simulink model "follower_v4"  (R2024a)
settings: Solver=VariableStepAuto  StartTime=0.0  StopTime=inf  RelTol=1e-6
values from neighbouring files (symbols this model uses):
  consigne = 0.6    [main.m]
undefined symbols (not defined in the file or in its folder): linear
libraries: ros2lib x5, slpidlib x1
settings Model: Creator=eswarm  LastModifiedBy=eswarm

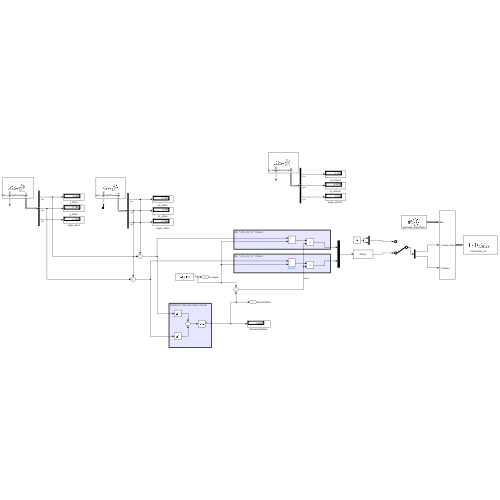
[thumbnail: Simulink's stored preview of the top-level diagram]
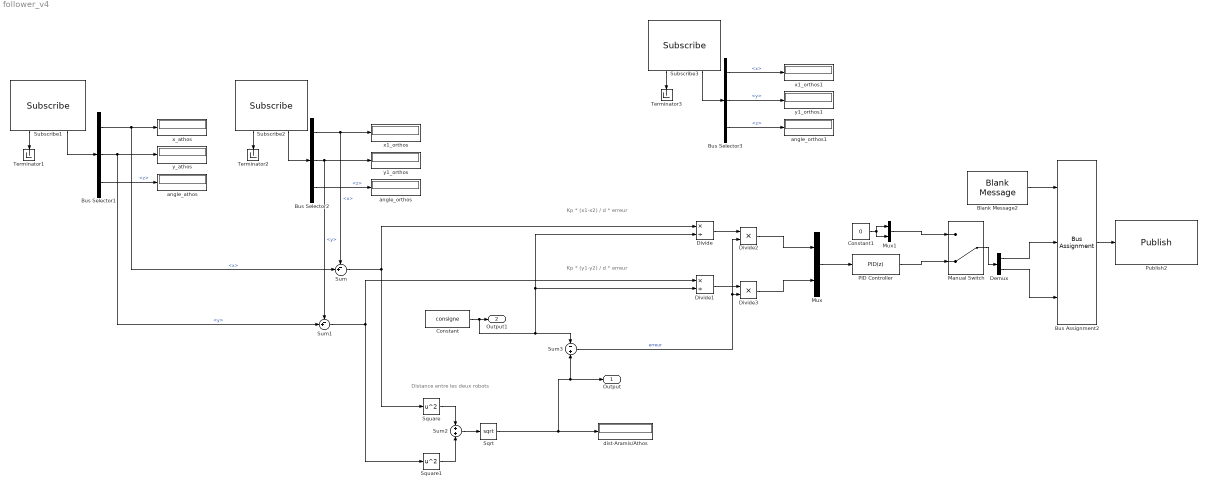
== system follower_v4 ==
  note: Distance entre les deux robots
  note: Kp * (x1-x2) / d * erreur
  note: Kp * (y1-y2) / d * erreur
  Blank Message2 : ros2lib/Blank Message  messageClass=Message  entityType=geometry_msgs/Twist  messageType=geometry_msgs/Twist  SampleTime=0.1
  Bus Assignment2 : BusAssignment  AssignedSignals=linear.x,linear.y
  Bus Selector1 : BusSelector  OutputSignals=pose.position.x,pose.position.y,pose.orientation.z
  Bus Selector2 : BusSelector  OutputSignals=pose.position.x,pose.position.y,pose.orientation.z
  Bus Selector3 : BusSelector  OutputSignals=pose.position.x,pose.position.y,pose.orientation.z
  Constant : Constant  Value=consigne
  Constant1 : Constant  Value=0
  Demux : Demux  Outputs=2
  Divide : Product  Inputs=*/  RndMeth=Zero  SaturateOnIntegerOverflow=on
  Divide1 : Product  Inputs=*/  RndMeth=Zero  SaturateOnIntegerOverflow=on
  Divide2 : Product  Inputs=**  RndMeth=Zero  SaturateOnIntegerOverflow=on
  Divide3 : Product  Inputs=**  RndMeth=Zero  SaturateOnIntegerOverflow=on
  Manual Switch : ManualSwitch  CurrentSetting=0
  Mux : Mux  Inputs=2
  Mux1 : Mux  Inputs=2
  PID Controller : slpidlib/PID Controller  Controller=PID  Form=Ideal  TimeDomain=Discrete-time  UseExternalTs=off  SampleTime=0.1  IntegratorMethod=Forward Euler  FilterMethod=Forward Euler  ControllerParametersSource=internal  P=0.5  I=0  UseKiTs=off  D=0  UseExternalDerivativeSource=off  N=100  UseFilter=on  TunerSelectOption=Transfer Function Based (PID Tuner App)  InitialConditionSource=internal  InitialConditionForIntegrator=0  InitialConditionForFilter=0  DifferentiatorICPrevScaledInput=0  ExternalReset=none  TrackingMode=off  Kt=1  LimitOutput=off  SatLimitsSource=internal  UpperSaturationLimit=inf  LowerSaturationLimit=-inf  LinearizeAsGain=on  AntiWindupMode=none  Kb=1  LimitIntegrator=off  UpperIntegratorSaturationLimit=inf  LowerIntegratorSaturationLimit=-inf  POutMin=[]  POutMax=[]  IOutMin=[]  IOutMax=[]  DOutMin=[]  DOutMax=[]  NOutMin=[]  NOutMax=[]  SumOutMin=[]  SumOutMax=[]  SaturationOutMin=[]  SaturationOutMax=[]  PParamMin=[]  PParamMax=[]  IParamMin=[]  IParamMax=[]  DParamMin=[]  DParamMax=[]  NParamMin=[]  NParamMax=[]  KbParamMin=[]  KbParamMax=[]  KtParamMin=[]  KtParamMax=[]  KbOutMin=[]  KbOutMax=[]  KtOutMin=[]  KtOutMax=[]  IntegratorOutMin=[]  IntegratorOutMax=[]  FilterOutMin=[]  FilterOutMax=[]  SumI1OutMin=[]  SumI1OutMax=[]  SumI2OutMin=[]  SumI2OutMax=[]  SumI3OutMin=[]  SumI3OutMax=[]  SumI4OutMin=[]  SumI4OutMax=[]  SumDOutMin=[]  SumDOutMax=[]  DifferentiatorOutMin=[]  DifferentiatorOutMax=[]  FilterDiffOutCoefMin=[]  FilterDiffOutCoefMax=[]  ReciprocalOutMin=[]  ReciprocalOutMax=[]  SumDenOutMin=[]  SumDenOutMax=[]  SumNumOutMin=[]  SumNumOutMax=[]  DivideOutMin=[]  DivideOutMax=[]  UdiffTsProdOutMin=[]  UdiffTsProdOutMax=[]  NTsProdOutMin=[]  NTsProdOutMax=[]  UintegralTsProdOutMin=[]  UintegralTsProdOutMax=[]  UngainTsProdOutMin=[]  UngainTsProdOutMax=[]  ClampingZeroOutDataTypeStr=Inherit: Inherit via back propagation  ClampingZeroOutMin=[]  ClampingZeroOutMax=[]  FilterDenConstantOutDataTypeStr=Inherit: Inherit via back propagation  FilterDenConstantOutMin=[]  FilterDenConstantOutMax=[]  PCopyOutDataTypeStr=Inherit: Inherit via back propagation  PCopyOutMin=[]  PCopyOutMax=[]  NCopyOutDataTypeStr=Inherit: Inherit via back propagation  NCopyOutMin=[]  NCopyOutMax=[]  IntegratorContinuousStateAttributes=''  IntegratorStateMustResolveToSignalObject=off  IntegratorRTWStateStorageClass=Auto  FilterContinuousStateAttributes=''  FilterStateMustResolveToSignalObject=off  FilterRTWStateStorageClass=Auto  ParallelPVariant=Passthrough  IdealPVariant=InternalParameters  IVariant=InternalParameters  DVariant=InternalParameters  IntegratorVariant=Discrete  SatVariant=Disabled  AWVariant=Passthrough  PCopyVariant=Disabled  TRVariant=Disabled  FdbkBlocksVariant=Forward  IdealPFdbkVariant=Disabled  SatFdbkVariant=Disabled  DerivativeFilterVariant=ForwardEulerFilter  NVariant=InternalParameters  NCopyVariant=Disabled  FilterICVariant=InternalICsFilter  IntegratorICVariant=InternalICs  ExternalResetVariant=Disabled  TRSumVariant=Passthrough  SumFdbkVariant=Disabled  SumVariant=Sum_PID  TsampFilterVariant=InternalTs  TsampNgainVariant=Passthrough  TsampIntegralVariant=Disabled_SignalSpec  ExternalSaturationOutDataTypeStr=Inherit: Same as second input  DerivativeSourceVariant=ErrorSignal
  Publish2 : ros2lib/Publish  topicSource=Select from ROS network  topic=/Athos/cmd_vel  messageType=geometry_msgs/Twist  QOSHistory=Keep last  QOSDepth=1  QOSReliability=Reliable  QOSDurability=Volatile  QOSDeadline=Inf  QOSLifespan=Inf  QOSLiveliness=Automatic  QOSLeaseDuration=Inf  QOSAvoidROSNamespaceConventions=off
  Sqrt : Sqrt
  Square : Math  Operator=square
  Square1 : Math  Operator=square
  Subscribe1 : ros2lib/Subscribe  topicSource=Select from ROS network  topic=/vrpn_mocap/Aramis/pose  messageType=geometry_msgs/PoseStamped  sampleTime=0.1  QOSHistory=Keep last  QOSDepth=1  QOSReliability=Reliable  QOSDurability=Volatile  QOSDeadline=Inf  QOSLifespan=Inf  QOSLiveliness=Automatic  QOSLeaseDuration=Inf  QOSAvoidROSNamespaceConventions=off
  Subscribe2 : ros2lib/Subscribe  topicSource=Select from ROS network  topic=/vrpn_mocap/Athos/pose  messageType=geometry_msgs/PoseStamped  sampleTime=0.1  QOSHistory=Keep last  QOSDepth=1  QOSReliability=Reliable  QOSDurability=Volatile  QOSDeadline=Inf  QOSLifespan=Inf  QOSLiveliness=Automatic  QOSLeaseDuration=Inf  QOSAvoidROSNamespaceConventions=off
  Subscribe3 : ros2lib/Subscribe  topicSource=Select from ROS network  topic=/vrpn_mocap/Porthos/pose  messageType=geometry_msgs/PoseStamped  sampleTime=0.1  QOSHistory=Keep last  QOSDepth=1  QOSReliability=Reliable  QOSDurability=Volatile  QOSDeadline=Inf  QOSLifespan=Inf  QOSLiveliness=Automatic  QOSLeaseDuration=Inf  QOSAvoidROSNamespaceConventions=off
  Sum : Sum  Inputs=-+|
  Sum1 : Sum  Inputs=-+|
  Sum2 : Sum  Inputs=+|+
  Sum3 : Sum  Inputs=-|+
  Terminator1 : Terminator
  Terminator2 : Terminator
  Terminator3 : Terminator
  angle_athos : Display
  angle_orthos : Display
  angle_orthos1 : Display
  dist-Aramis/Athos : Display
  x1_orthos : Display
  x1_orthos1 : Display
  x_athos : Display
  y1_orthos : Display
  y1_orthos1 : Display
  y_athos : Display
  Output : Outport  SignalName=Aramis/Athos
  Output1 : Outport  Port=2  SignalName=consigne
  wires:
  Bus Selector1/1 -> Sum/2, x_athos/1  "<x>"
  Subscribe2/1 -> Terminator2/1
  Bus Selector2/2 -> Sum1/1, y1_orthos/1  "<y>"
  Bus Selector2/3 -> angle_orthos/1  "<z>"
  Subscribe1/2 -> Bus Selector1/1
  Bus Selector1/3 -> angle_athos/1  "<z>"
  Bus Selector1/2 -> Sum1/2, y_athos/1  "<y>"
  Bus Selector2/1 -> Sum/1, x1_orthos/1  "<x>"
  Subscribe1/1 -> Terminator1/1
  Subscribe2/2 -> Bus Selector2/1
  Subscribe3/2 -> Bus Selector3/1
  Bus Selector3/1 -> x1_orthos1/1  "<x>"
  Bus Selector3/3 -> angle_orthos1/1  "<z>"
  Subscribe3/1 -> Terminator3/1
  Bus Selector3/2 -> y1_orthos1/1  "<y>"
  Square/1 -> Sum2/1
  Square1/1 -> Sum2/2
  Sum2/1 -> Sqrt/1
  Sqrt/1 -> Sum3/2, Output/1, dist-Aramis/Athos/1
  Constant/1 -> Divide/2, Divide1/2, Sum3/1, Output1/1
  Divide3/1 -> Mux/2
  Sum/1 -> Divide/1, Square/1
  Sum1/1 -> Square1/1, Divide1/1
  Divide1/1 -> Divide3/1
  Divide/1 -> Divide2/1
  Sum3/1 -> Divide2/2, Divide3/2  "erreur"
  Divide2/1 -> Mux/1
  Bus Assignment2/1 -> Publish2/1
  Blank Message2/1 -> Bus Assignment2/1
  Mux/1 -> PID Controller/1
  Demux/1 -> Bus Assignment2/2
  Demux/2 -> Bus Assignment2/3
  Constant1/1 -> Mux1/1, Mux1/2
  Manual Switch/1 -> Demux/1
  PID Controller/1 -> Manual Switch/2
  Mux1/1 -> Manual Switch/1
